simulink model "sampleModel7126_pp_1_1"  (R2018a)
settings: Solver=VariableStepAuto  StartTime=0.0  StopTime=10.0  RelTol=1e-3
undefined symbols (not defined in the file): DiscIntNeverNeededParam
libraries: simulink x367
(part 3 of 12)

== system sampleModel7126_pp_1_1/cfblk256 ==
  cfblk1 : Inport
  cfblk10 : Inport  Port=2
  Action Port : ActionPort  ActionType=else
  cfblk11 : Subsystem  TreatAsAtomicUnit=on
  cfblk12 : Subsystem  TreatAsAtomicUnit=on
  cfblk13 : Delay
  cfblk14 : Subsystem  TreatAsAtomicUnit=on
  cfblk15 : Delay
  cfblk3 : Subsystem  TreatAsAtomicUnit=on
  cfblk4 : DiscreteStateSpace  SampleTime=-1
  cfblk5 : DiscreteTransferFcn
  cfblk6 : simulink/Discrete/Transfer Fcn Real Zero  ZeroZ=0.75  ICPrevInput=0.0  DoSatur=off
      settings: SourceProductName=Simulink  SourceProductBaseCode=SL
  cfblk7 : simulink/Continuous/PID Controller  Controller=PID  TimeDomain=Discrete-time  SampleTime=-1  IntegratorMethod=Forward Euler  FilterMethod=Forward Euler  Form=Parallel  UseFilter=on  ControllerParametersSource=internal  P=1  I=1  D=0  N=100  InitialConditionSource=internal  InitialConditionForIntegrator=0  InitialConditionForFilter=0  ExternalReset=none  LimitOutput=off  UpperSaturationLimit=inf  LowerSaturationLimit=-inf  LinearizeAsGain=off  AntiWindupMode=none  Kb=1  TrackingMode=off  Kt=1  PParamMin=[]  PParamMax=[]  IParamMin=[]  IParamMax=[]  DParamMin=[]  DParamMax=[]  NParamMin=[]  NParamMax=[]  KbParamMin=[]  KbParamMax=[]  KtParamMin=[]  KtParamMax=[]  POutMin=[]  POutMax=[]  IOutMin=[]  IOutMax=[]  DOutMin=[]  DOutMax=[]  NOutMin=[]  NOutMax=[]  KbOutMin=[]  KbOutMax=[]  KtOutMin=[]  KtOutMax=[]  IntegratorOutMin=[]  IntegratorOutMax=[]  FilterOutMin=[]  FilterOutMax=[]  SumOutMin=[]  SumOutMax=[]  SumI1OutMin=[]  SumI1OutMax=[]  SumI2OutMin=[]  SumI2OutMax=[]  SumI3OutMin=[]  SumI3OutMax=[]  SumDOutMin=[]  SumDOutMax=[]  SaturationOutMin=[]  SaturationOutMax=[]  IntegratorContinuousStateAttributes=''  IntegratorStateMustResolveToSignalObject=off  IntegratorRTWStateStorageClass=Auto  FilterContinuousStateAttributes=''  FilterStateMustResolveToSignalObject=off  FilterRTWStateStorageClass=Auto  DifferentiatorICPrevScaledInput=0  DifferentiatorOutMin=[]  DifferentiatorOutMax=[]  FilterDiffOutCoefMin=[]  FilterDiffOutCoefMax=[]  SumDenOutMin=[]  SumDenOutMax=[]  SumNumOutMin=[]  SumNumOutMax=[]  ReciprocalOutMin=[]  ReciprocalOutMax=[]  DivideOutMin=[]  DivideOutMax=[]  TunerSelectOption=Transfer Function Based (PID Tuner App)
  cfblk8 : DiscreteFir
  cfblk9 : If  SampleTime=1
  cyemi_{359..361,368,373..382} (14 alike) : DataTypeConversion  OutDataTypeStr=double
  emi_1040 : Subsystem  TreatAsAtomicUnit=on
  emi_1042 : If  IfExpression=0 <= u1  SampleTime=[1 0]
  emi_1043 : DataTypeConversion  OutDataTypeStr=double
  emi_2146 : Subsystem  TreatAsAtomicUnit=on
  emi_2148 : If  IfExpression=0 <= u1  SampleTime=[1 0]
  emi_2149 : DataTypeConversion  OutDataTypeStr=double
  cfblk2 : Outport
  wires:
  cfblk1/1 -> cfblk2/1
  cfblk9/1 -> cfblk11/Action
  cfblk9/2 -> cfblk12/Action
  cyemi_359/1 -> cfblk11/1(cfblk1)
  cfblk13/1 -> cyemi_359/1, emi_1043/1
  cyemi_360/1 -> cfblk11/2(cfblk9)
  cfblk10/1 -> cyemi_360/1
  cyemi_361/1 -> cfblk11/3(cfblk10)
  cfblk12/3(cfblk8) -> cyemi_361/1
  cyemi_368/1 -> cfblk12/1(cfblk1)
  cfblk6/1 -> cyemi_368/1
  cyemi_373/1 -> cfblk13/1
  cfblk4/1 -> cyemi_373/1
  cfblk12/1(cfblk2) -> cyemi_374/1
  cyemi_375/1 -> cfblk15/1
  cfblk12/2(cfblk7) -> cyemi_375/1
  cfblk15/1 -> cyemi_376/1
  cyemi_377/1 -> cfblk4/1
  cfblk8/1 -> cyemi_377/1
  cyemi_378/1 -> cfblk5/1
  cfblk7/1 -> cyemi_378/1
  cyemi_379/1 -> cfblk6/1
  cfblk5/1 -> cyemi_379/1
  cyemi_380/1 -> cfblk7/1
  cyemi_381/1 -> cfblk8/1
  cfblk11/1(cfblk2) -> cyemi_381/1
  cyemi_382/1 -> cfblk9/1
  cyemi_376/1 -> cfblk3/1(emi_1038)
  cfblk3/1(emi_1039) -> cyemi_380/1, emi_2149/1
  emi_1042/1 -> cfblk3/Action
  emi_1042/2 -> emi_1040/Action
  emi_1043/1 -> emi_1042/1
  cyemi_374/1 -> cfblk14/1(emi_2144)
  cfblk14/1(emi_2145) -> cyemi_382/1
  emi_2148/1 -> cfblk14/Action
  emi_2148/2 -> emi_2146/Action
  emi_2149/1 -> emi_2148/1

== system sampleModel7126_pp_1_1/cfblk257 ==
  cfblk1 : Inport
  cfblk12 : Inport  Port=2
  cfblk13 : Inport  Port=3
  Action Port : ActionPort  ActionType=then
  cfblk10 : simulink/Discrete/Tapped Delay  vinit=0.0  samptime=-1  NumDelays=1  DelayOrder=Oldest  includeCurrent=off
  cfblk11 : simulink/Discrete/Difference  ICPrevInput=0.0  OutMin=[]  OutMax=[]  OutDataTypeStr=double  OutputDataTypeScalingMode=double  OutDataType=fixdt(1, 16)  OutScaling=2^-10  DoSatur=off
  cfblk3 : DiscreteFir
  cfblk4 : simulink/Continuous/PID Controller  Controller=PID  TimeDomain=Discrete-time  SampleTime=-1  IntegratorMethod=Forward Euler  FilterMethod=Forward Euler  Form=Parallel  UseFilter=on  ControllerParametersSource=internal  P=1  I=1  D=0  N=100  InitialConditionSource=internal  InitialConditionForIntegrator=0  InitialConditionForFilter=0  ExternalReset=none  LimitOutput=off  UpperSaturationLimit=inf  LowerSaturationLimit=-inf  LinearizeAsGain=off  AntiWindupMode=none  Kb=1  TrackingMode=off  Kt=1  PParamMin=[]  PParamMax=[]  IParamMin=[]  IParamMax=[]  DParamMin=[]  DParamMax=[]  NParamMin=[]  NParamMax=[]  KbParamMin=[]  KbParamMax=[]  KtParamMin=[]  KtParamMax=[]  POutMin=[]  POutMax=[]  IOutMin=[]  IOutMax=[]  DOutMin=[]  DOutMax=[]  NOutMin=[]  NOutMax=[]  KbOutMin=[]  KbOutMax=[]  KtOutMin=[]  KtOutMax=[]  IntegratorOutMin=[]  IntegratorOutMax=[]  FilterOutMin=[]  FilterOutMax=[]  SumOutMin=[]  SumOutMax=[]  SumI1OutMin=[]  SumI1OutMax=[]  SumI2OutMin=[]  SumI2OutMax=[]  SumI3OutMin=[]  SumI3OutMax=[]  SumDOutMin=[]  SumDOutMax=[]  SaturationOutMin=[]  SaturationOutMax=[]  IntegratorContinuousStateAttributes=''  IntegratorStateMustResolveToSignalObject=off  IntegratorRTWStateStorageClass=Auto  FilterContinuousStateAttributes=''  FilterStateMustResolveToSignalObject=off  FilterRTWStateStorageClass=Auto  DifferentiatorICPrevScaledInput=0  DifferentiatorOutMin=[]  DifferentiatorOutMax=[]  FilterDiffOutCoefMin=[]  FilterDiffOutCoefMax=[]  SumDenOutMin=[]  SumDenOutMax=[]  SumNumOutMin=[]  SumNumOutMax=[]  ReciprocalOutMin=[]  ReciprocalOutMax=[]  DivideOutMin=[]  DivideOutMax=[]  TunerSelectOption=Transfer Function Based (PID Tuner App)
  cfblk5 : simulink/Discrete/Transfer Fcn Real Zero  ZeroZ=0.75  ICPrevInput=0.0  DoSatur=off
      settings: SourceProductName=Simulink  SourceProductBaseCode=SL
  cfblk6 : simulink/Continuous/PID Controller  Controller=PID  TimeDomain=Discrete-time  SampleTime=-1  IntegratorMethod=Forward Euler  FilterMethod=Forward Euler  Form=Parallel  UseFilter=on  ControllerParametersSource=internal  P=1  I=1  D=0  N=100  InitialConditionSource=internal  InitialConditionForIntegrator=0  InitialConditionForFilter=0  ExternalReset=none  LimitOutput=off  UpperSaturationLimit=inf  LowerSaturationLimit=-inf  LinearizeAsGain=off  AntiWindupMode=none  Kb=1  TrackingMode=off  Kt=1  PParamMin=[]  PParamMax=[]  IParamMin=[]  IParamMax=[]  DParamMin=[]  DParamMax=[]  NParamMin=[]  NParamMax=[]  KbParamMin=[]  KbParamMax=[]  KtParamMin=[]  KtParamMax=[]  POutMin=[]  POutMax=[]  IOutMin=[]  IOutMax=[]  DOutMin=[]  DOutMax=[]  NOutMin=[]  NOutMax=[]  KbOutMin=[]  KbOutMax=[]  KtOutMin=[]  KtOutMax=[]  IntegratorOutMin=[]  IntegratorOutMax=[]  FilterOutMin=[]  FilterOutMax=[]  SumOutMin=[]  SumOutMax=[]  SumI1OutMin=[]  SumI1OutMax=[]  SumI2OutMin=[]  SumI2OutMax=[]  SumI3OutMin=[]  SumI3OutMax=[]  SumDOutMin=[]  SumDOutMax=[]  SaturationOutMin=[]  SaturationOutMax=[]  IntegratorContinuousStateAttributes=''  IntegratorStateMustResolveToSignalObject=off  IntegratorRTWStateStorageClass=Auto  FilterContinuousStateAttributes=''  FilterStateMustResolveToSignalObject=off  FilterRTWStateStorageClass=Auto  DifferentiatorICPrevScaledInput=0  DifferentiatorOutMin=[]  DifferentiatorOutMax=[]  FilterDiffOutCoefMin=[]  FilterDiffOutCoefMax=[]  SumDenOutMin=[]  SumDenOutMax=[]  SumNumOutMin=[]  SumNumOutMax=[]  ReciprocalOutMin=[]  ReciprocalOutMax=[]  DivideOutMin=[]  DivideOutMax=[]  TunerSelectOption=Transfer Function Based (PID Tuner App)
  cfblk7 : Subsystem  TreatAsAtomicUnit=on
  cfblk8 : UnitDelay  SampleTime=-1
  cfblk9 : Subsystem  TreatAsAtomicUnit=on
  cyemi_{386..394} (9 alike) : DataTypeConversion  OutDataTypeStr=double
  emi_1634 : Subsystem  TreatAsAtomicUnit=on
  emi_1636 : If  IfExpression=Inf <= u1  SampleTime=[1 0]
  emi_1637 : DataTypeConversion  OutDataTypeStr=double
  emi_727 : Subsystem  TreatAsAtomicUnit=on
  emi_729 : If  IfExpression=Inf <= u1  SampleTime=[1 0]
  emi_730 : DataTypeConversion  OutDataTypeStr=double
  cfblk2 : Outport
  cfblk14 : Outport  Port=2
  wires:
  cfblk3/1 -> cfblk14/1, emi_730/1
  cfblk11/1 -> cfblk2/1
  cyemi_386/1 -> cfblk10/1
  cfblk1/1 -> cyemi_386/1
  cyemi_387/1 -> cfblk11/1
  cfblk6/1 -> cyemi_387/1
  cyemi_388/1 -> cfblk3/1
  cfblk8/1 -> cyemi_388/1
  cyemi_389/1 -> cfblk4/1
  cfblk12/1 -> cyemi_389/1
  cyemi_390/1 -> cfblk5/1
  cyemi_391/1 -> cfblk6/1
  cfblk4/1 -> cyemi_392/1
  cyemi_393/1 -> cfblk8/1
  cfblk5/1 -> cyemi_393/1
  cfblk10/1 -> cyemi_394/1, emi_1637/1
  cyemi_394/1 -> cfblk9/1(emi_725)
  cfblk9/1(emi_726) -> cyemi_391/1
  emi_729/1 -> cfblk9/Action
  emi_729/2 -> emi_727/Action
  emi_730/1 -> emi_729/1
  cyemi_392/1 -> cfblk7/1(emi_1632)
  cfblk7/1(emi_1633) -> cyemi_390/1
  emi_1636/1 -> cfblk7/Action
  emi_1636/2 -> emi_1634/Action
  emi_1637/1 -> emi_1636/1

== system sampleModel7126_pp_1_1/cfblk258 ==
  cfblk1 : Inport
  cfblk8 : Inport  Port=2
  cfblk9 : Inport  Port=3
  cfblk10 : Inport  Port=4
  Action Port : ActionPort  ActionType=else
  cfblk11 : Delay
  cfblk3 : UnitDelay  SampleTime=-1
  cfblk4 : DiscreteFir
  cfblk5 : Subsystem  TreatAsAtomicUnit=on
  cfblk6 : Delay  ShowEnablePort=on
      settings: InputPortMap=u0,e6
  cfblk7 : simulink/Continuous/PID Controller (2DOF)  Controller=PID  TimeDomain=Discrete-time  SampleTime=-1  IntegratorMethod=Forward Euler  FilterMethod=Forward Euler  Form=Parallel  UseFilter=on  ControllerParametersSource=internal  P=1  I=1  D=0  N=100  b=1  c=1  InitialConditionSource=internal  InitialConditionForIntegrator=0  InitialConditionForFilter=0  ExternalReset=none  LimitOutput=off  UpperSaturationLimit=inf  LowerSaturationLimit=-inf  LinearizeAsGain=off  AntiWindupMode=none  Kb=1  TrackingMode=off  Kt=1  PParamMin=[]  PParamMax=[]  IParamMin=[]  IParamMax=[]  DParamMin=[]  DParamMax=[]  NParamMin=[]  NParamMax=[]  bParamMin=[]  bParamMax=[]  cParamMin=[]  cParamMax=[]  KbParamMin=[]  KbParamMax=[]  KtParamMin=[]  KtParamMax=[]  POutMin=[]  POutMax=[]  IOutMin=[]  IOutMax=[]  DOutMin=[]  DOutMax=[]  NOutMin=[]  NOutMax=[]  bOutMin=[]  bOutMax=[]  cOutMin=[]  cOutMax=[]  KbOutMin=[]  KbOutMax=[]  KtOutMin=[]  KtOutMax=[]  IntegratorOutMin=[]  IntegratorOutMax=[]  FilterOutMin=[]  FilterOutMax=[]  SumOutMin=[]  SumOutMax=[]  Sum1OutMin=[]  Sum1OutMax=[]  Sum2OutMin=[]  Sum2OutMax=[]  Sum3OutMin=[]  Sum3OutMax=[]  SumI1OutMin=[]  SumI1OutMax=[]  SumI2OutMin=[]  SumI2OutMax=[]  SumI3OutMin=[]  SumI3OutMax=[]  SumDOutMin=[]  SumDOutMax=[]  SaturationOutMin=[]  SaturationOutMax=[]  IntegratorContinuousStateAttributes=''  IntegratorStateMustResolveToSignalObject=off  IntegratorRTWStateStorageClass=Auto  FilterContinuousStateAttributes=''  FilterStateMustResolveToSignalObject=off  FilterRTWStateStorageClass=Auto  DifferentiatorICPrevScaledInput=0  DifferentiatorOutMin=[]  DifferentiatorOutMax=[]  FilterDiffOutCoefMin=[]  FilterDiffOutCoefMax=[]  SumDenOutMin=[]  SumDenOutMax=[]  SumNumOutMin=[]  SumNumOutMax=[]  ReciprocalOutMin=[]  ReciprocalOutMax=[]  DivideOutMin=[]  DivideOutMax=[]  TunerSelectOption=Transfer Function Based (PID Tuner App)
  cyemi_{399..406} (8 alike) : DataTypeConversion  OutDataTypeStr=double
  emi_1343 : Subsystem  TreatAsAtomicUnit=on
  emi_1345 : If  IfExpression=0 <= u1  SampleTime=[1 0]
  emi_1346 : DataTypeConversion  OutDataTypeStr=double
  cfblk2 : Outport
  wires:
  cfblk10/1 -> cfblk2/1
  cyemi_399/1 -> cfblk11/1
  cyemi_400/1 -> cfblk3/1
  cfblk9/1 -> cyemi_400/1
  cyemi_401/1 -> cfblk4/1
  cfblk8/1 -> cyemi_401/1
  cfblk7/1 -> cyemi_402/1
  cyemi_403/1 -> cfblk6/1
  cfblk11/1 -> cyemi_403/1
  cyemi_404/1 -> cfblk6/2
  cfblk3/1 -> cyemi_404/1, emi_1346/1
  cyemi_405/1 -> cfblk7/1
  cfblk4/1 -> cyemi_405/1
  cyemi_406/1 -> cfblk7/2
  cfblk6/1 -> cyemi_406/1
  cyemi_402/1 -> cfblk5/1(emi_1341)
  cfblk5/1(emi_1342) -> cyemi_399/1
  emi_1345/1 -> cfblk5/Action
  emi_1345/2 -> emi_1343/Action
  emi_1346/1 -> emi_1345/1

== system sampleModel7126_pp_1_1/cfblk259 ==
  cfblk1 : Inport
  Action Port : ActionPort  ActionType=then
  cfblk10 : Subsystem  TreatAsAtomicUnit=on
  cfblk11 : Subsystem  TreatAsAtomicUnit=on
  cfblk12 : Delay
  cfblk13 : Subsystem  TreatAsAtomicUnit=on
  cfblk3 : Subsystem  TreatAsAtomicUnit=on
  cfblk4 : Subsystem  TreatAsAtomicUnit=on
  cfblk5 : simulink/Discrete/Tapped Delay  vinit=0.0  samptime=-1  NumDelays=1  DelayOrder=Oldest  includeCurrent=off
  cfblk6 : Subsystem  TreatAsAtomicUnit=on
  cfblk7 : If  SampleTime=1
  cfblk9 : Subsystem  TreatAsAtomicUnit=on
  cyemi_{408..411,421..431} (15 alike) : DataTypeConversion  OutDataTypeStr=double
  emi_1161 : Subsystem  TreatAsAtomicUnit=on
  emi_{62,560,1163,1774} (4 alike) : If  IfExpression=Inf <= u1  SampleTime=[1 0]
  emi_{48,63,561,1164,1775} (5 alike) : DataTypeConversion  OutDataTypeStr=double
  emi_1772 : Subsystem  TreatAsAtomicUnit=on
  emi_45 : Subsystem  TreatAsAtomicUnit=on
  emi_47 : If  IfExpression=Inf <= u1
  emi_558 : Subsystem  TreatAsAtomicUnit=on
  emi_60 : Subsystem  TreatAsAtomicUnit=on
  cfblk2 : Outport
  cfblk8 : Outport  Port=2
  wires:
  cfblk5/1 -> cfblk8/1, cyemi_421/1, emi_63/1, emi_1775/1
  cfblk7/1 -> cfblk9/Action
  cfblk7/2 -> cfblk10/Action
  cyemi_408/1 -> cfblk10/1(cfblk1)
  cfblk1/1 -> cyemi_408/1
  cyemi_409/1 -> cfblk10/2(cfblk10)
  cyemi_410/1 -> cfblk10/3(cfblk11)
  cyemi_411/1 -> cfblk10/4(cfblk12)
  cyemi_422/1 -> cfblk12/1
  cfblk9/1(cfblk2) -> cyemi_422/1
  cfblk9/2(cfblk12) -> cyemi_423/1
  cfblk9/3(cfblk13) -> cyemi_424/1, cyemi_425/1
  cyemi_427/1 -> cfblk5/1
  cfblk10/1(cfblk2) -> cyemi_427/1
  cyemi_429/1 -> cfblk7/1
  cfblk12/1 -> cyemi_429/1
  cyemi_430/1 -> cfblk9/1(cfblk1)
  cyemi_431/1 -> cfblk9/2(cfblk11)
  cyemi_421/1 -> cfblk11/1(emi_43)
  cfblk11/1(emi_44) -> cyemi_411/1, emi_561/1, emi_1164/1
  emi_47/1 -> cfblk11/Action
  emi_47/2 -> emi_45/Action
  emi_48/1 -> emi_47/1
  cyemi_423/1 -> cfblk13/1(emi_58)
  cfblk13/1(emi_59) -> cyemi_428/1
  emi_62/1 -> cfblk13/Action
  emi_62/2 -> emi_60/Action
  emi_63/1 -> emi_62/1
  cyemi_428/1 -> cfblk6/1(emi_556)
  cfblk6/1(emi_557) -> cyemi_431/1, cyemi_430/1, cyemi_426/1, cyemi_410/1
  emi_560/1 -> cfblk6/Action
  emi_560/2 -> emi_558/Action
  emi_561/1 -> emi_560/1
  cyemi_426/1 -> cfblk4/1(emi_1159)
  cfblk4/1(emi_1160) -> emi_48/1, cyemi_409/1
  emi_1163/1 -> cfblk4/Action
  emi_1163/2 -> emi_1161/Action
  emi_1164/1 -> emi_1163/1
  cyemi_424/1 -> cfblk3/1(emi_1769)
  cyemi_425/1 -> cfblk3/2(emi_1770)
  cfblk3/1(emi_1771) -> cfblk2/1
  emi_1774/1 -> cfblk3/Action
  emi_1774/2 -> emi_1772/Action
  emi_1775/1 -> emi_1774/1

== system sampleModel7126_pp_1_1/cfblk26 ==
  emi_1504 : Inport
  Action Port : ActionPort  ActionType=then
  cfblk26 : simulink/Discrete/Transfer Fcn First Order  PoleZ=0.95  ICPrevOutput=0.0  DoSatur=off
      settings: SourceProductName=Simulink
  emi_1505 : Outport
  wires:
  emi_1504/1 -> cfblk26/1
  cfblk26/1 -> emi_1505/1

== system sampleModel7126_pp_1_1/cfblk260 ==
  cfblk1 : Inport
  cfblk9 : Inport  Port=2
  Action Port : ActionPort  ActionType=else
  cfblk13 : Delay
  cfblk3 : simulink/Discrete/Transfer Fcn Real Zero  ZeroZ=0.75  ICPrevInput=0.0  DoSatur=off
      settings: SourceProductName=Simulink  SourceProductBaseCode=SL
  cfblk4 : Subsystem  TreatAsAtomicUnit=on
  cfblk5 : Subsystem  TreatAsAtomicUnit=on
  cfblk6 : Subsystem  TreatAsAtomicUnit=on
  cfblk7 : Delay  DelayLengthSource=Input port
      settings: InputPortMap=u0,p1
  cfblk8 : simulink/Discrete/Transfer Fcn Lead or Lag  PoleZ=0.95  ZeroZ=0.75  ICPrevOutput=0.0  ICPrevInput=0.0  DoSatur=off
      settings: SourceProductName=Simulink  SourceProductBaseCode=SL
  cyemi_{449..456} (8 alike) : DataTypeConversion  OutDataTypeStr=double
  emi_10 : Subsystem  TreatAsAtomicUnit=on
  emi_12 : If  IfExpression=0 <= u1  SampleTime=[1 0]
  emi_13 : DataTypeConversion  OutDataTypeStr=double
  emi_254 : Subsystem  TreatAsAtomicUnit=on
  emi_256 : If  IfExpression=0 <= u1  SampleTime=[1 0]
  emi_257 : DataTypeConversion  OutDataTypeStr=double
  emi_410 : Subsystem  TreatAsAtomicUnit=on
  emi_412 : If  IfExpression=0 <= u1  SampleTime=[1 0]
  emi_413 : DataTypeConversion  OutDataTypeStr=double
  cfblk2 : Outport
  cfblk10 : Outport  Port=2
  cfblk11 : Outport  Port=3
  cfblk12 : Outport  Port=4
  wires:
  cfblk8/1 -> cfblk10/1
  cfblk3/1 -> cyemi_451/1, cyemi_452/1
  cfblk9/1 -> cfblk11/1, cfblk2/1
  cyemi_449/1 -> cfblk13/1
  cyemi_450/1 -> cfblk3/1
  cfblk13/1 -> cyemi_450/1, emi_13/1, emi_257/1
  cyemi_454/1 -> cfblk7/1
  cyemi_455/1 -> cfblk7/2
  cfblk1/1 -> cyemi_455/1
  cyemi_456/1 -> cfblk8/1
  cfblk7/1 -> cyemi_456/1
  cyemi_452/1 -> cfblk5/1(emi_8)
  cfblk5/1(emi_9) -> cyemi_449/1, emi_413/1
  emi_12/1 -> cfblk5/Action
  emi_12/2 -> emi_10/Action
  emi_13/1 -> emi_12/1
  cyemi_451/1 -> cfblk4/1(emi_252)
  cfblk4/1(emi_253) -> cyemi_453/1, cfblk12/1
  emi_256/1 -> cfblk4/Action
  emi_256/2 -> emi_254/Action
  emi_257/1 -> emi_256/1
  cyemi_453/1 -> cfblk6/1(emi_408)
  cfblk6/1(emi_409) -> cyemi_454/1
  emi_412/1 -> cfblk6/Action
  emi_412/2 -> emi_410/Action
  emi_413/1 -> emi_412/1

== system sampleModel7126_pp_1_1/cfblk261 ==
  cfblk1 : Inport
  Action Port : ActionPort  ActionType=then
  cfblk10 : simulink/Discrete/Difference  ICPrevInput=0.0  OutMin=[]  OutMax=[]  OutDataTypeStr=double  OutputDataTypeScalingMode=double  OutDataType=fixdt(1, 16)  OutScaling=2^-10  DoSatur=off
  cfblk11 : If  SampleTime=1
  cfblk13 : Subsystem  TreatAsAtomicUnit=on
  cfblk14 : Subsystem  TreatAsAtomicUnit=on
  cfblk15 : Subsystem  TreatAsAtomicUnit=on
  cfblk16 : Delay
  cfblk17 : Delay
  cfblk3 : simulink/Discrete/Difference  ICPrevInput=0.0  OutMin=[]  OutMax=[]  OutDataTypeStr=double  OutputDataTypeScalingMode=double  OutDataType=fixdt(1, 16)  OutScaling=2^-10  DoSatur=off
  cfblk4 : DiscreteFilter
  cfblk5 : DiscreteTransferFcn
  cfblk6 : simulink/Continuous/PID Controller (2DOF)  Controller=PID  TimeDomain=Discrete-time  SampleTime=-1  IntegratorMethod=Forward Euler  FilterMethod=Forward Euler  Form=Parallel  UseFilter=on  ControllerParametersSource=internal  P=1  I=1  D=0  N=100  b=1  c=1  InitialConditionSource=internal  InitialConditionForIntegrator=0  InitialConditionForFilter=0  ExternalReset=none  LimitOutput=off  UpperSaturationLimit=inf  LowerSaturationLimit=-inf  LinearizeAsGain=off  AntiWindupMode=none  Kb=1  TrackingMode=off  Kt=1  PParamMin=[]  PParamMax=[]  IParamMin=[]  IParamMax=[]  DParamMin=[]  DParamMax=[]  NParamMin=[]  NParamMax=[]  bParamMin=[]  bParamMax=[]  cParamMin=[]  cParamMax=[]  KbParamMin=[]  KbParamMax=[]  KtParamMin=[]  KtParamMax=[]  POutMin=[]  POutMax=[]  IOutMin=[]  IOutMax=[]  DOutMin=[]  DOutMax=[]  NOutMin=[]  NOutMax=[]  bOutMin=[]  bOutMax=[]  cOutMin=[]  cOutMax=[]  KbOutMin=[]  KbOutMax=[]  KtOutMin=[]  KtOutMax=[]  IntegratorOutMin=[]  IntegratorOutMax=[]  FilterOutMin=[]  FilterOutMax=[]  SumOutMin=[]  SumOutMax=[]  Sum1OutMin=[]  Sum1OutMax=[]  Sum2OutMin=[]  Sum2OutMax=[]  Sum3OutMin=[]  Sum3OutMax=[]  SumI1OutMin=[]  SumI1OutMax=[]  SumI2OutMin=[]  SumI2OutMax=[]  SumI3OutMin=[]  SumI3OutMax=[]  SumDOutMin=[]  SumDOutMax=[]  SaturationOutMin=[]  SaturationOutMax=[]  IntegratorContinuousStateAttributes=''  IntegratorStateMustResolveToSignalObject=off  IntegratorRTWStateStorageClass=Auto  FilterContinuousStateAttributes=''  FilterStateMustResolveToSignalObject=off  FilterRTWStateStorageClass=Auto  DifferentiatorICPrevScaledInput=0  DifferentiatorOutMin=[]  DifferentiatorOutMax=[]  FilterDiffOutCoefMin=[]  FilterDiffOutCoefMax=[]  SumDenOutMin=[]  SumDenOutMax=[]  SumNumOutMin=[]  SumNumOutMax=[]  ReciprocalOutMin=[]  ReciprocalOutMax=[]  DivideOutMin=[]  DivideOutMax=[]  TunerSelectOption=Transfer Function Based (PID Tuner App)
  cfblk7 : Delay  ShowEnablePort=on
      settings: InputPortMap=u0,e6
  cfblk8 : Subsystem  TreatAsAtomicUnit=on
  cfblk9 : Subsystem  TreatAsAtomicUnit=on
  cyemi_{458..460,469..470,473..484} (17 alike) : DataTypeConversion  OutDataTypeStr=double
  emi_1966 : Subsystem  TreatAsAtomicUnit=on
  emi_1968 : If  IfExpression=0 <= u1  SampleTime=[1 0]
  emi_1969 : DataTypeConversion  OutDataTypeStr=double
  emi_1973 : Subsystem  TreatAsAtomicUnit=on
  emi_1975 : If  IfExpression=0 <= u1  SampleTime=[1 0]
  emi_1976 : DataTypeConversion  OutDataTypeStr=double
  emi_2196 : Subsystem  TreatAsAtomicUnit=on
  emi_2198 : If  IfExpression=0 <= u1  SampleTime=[0.1 0]
  emi_2199 : DataTypeConversion  OutDataTypeStr=double
  cfblk2 : Outport
  cfblk12 : Outport  Port=2
  wires:
  cfblk7/1 -> cyemi_459/1, cyemi_476/1
  cfblk13/1(cfblk2) -> cyemi_470/1, cyemi_479/1
  cfblk14/1(cfblk2) -> cfblk12/1
  cfblk11/1 -> cfblk13/Action
  cfblk11/2 -> cfblk14/Action
  cyemi_458/1 -> cfblk10/1
  cfblk14/3(cfblk7) -> cyemi_458/1
  cyemi_459/1 -> cfblk11/1
  cyemi_460/1 -> cfblk13/1(cfblk1)
  cfblk3/1 -> cyemi_460/1
  cyemi_469/1 -> cfblk14/1(cfblk1)
  cfblk16/1 -> cyemi_469/1
  cyemi_470/1 -> cfblk14/2(cfblk5)
  cyemi_474/1 -> cfblk16/1
  cfblk4/1 -> cyemi_474/1, emi_1969/1, emi_1976/1, emi_2199/1
  cyemi_475/1 -> cfblk17/1
  cfblk10/1 -> cyemi_475/1
  cyemi_476/1 -> cfblk3/1
  cyemi_477/1 -> cfblk4/1
  cfblk14/2(cfblk6) -> cyemi_477/1
  cyemi_478/1 -> cfblk5/1
  cyemi_479/1 -> cfblk6/1
  cyemi_480/1 -> cfblk6/2
  cyemi_481/1 -> cfblk7/1
  cfblk1/1 -> cyemi_481/1
  cyemi_482/1 -> cfblk7/2
  cfblk17/1 -> cyemi_482/1
  cfblk6/1 -> cyemi_483/1
  cfblk5/1 -> cyemi_484/1
  cyemi_473/1 -> cfblk15/1(emi_1964)
  cfblk15/1(emi_1965) -> cyemi_480/1
  emi_1968/1 -> cfblk15/Action
  emi_1968/2 -> emi_1966/Action
  emi_1969/1 -> emi_1968/1
  cyemi_483/1 -> cfblk8/1(emi_1971)
  cfblk8/1(emi_1972) -> cyemi_478/1, cyemi_473/1
  emi_1975/1 -> cfblk8/Action
  emi_1975/2 -> emi_1973/Action
  emi_1976/1 -> emi_1975/1
  cyemi_484/1 -> cfblk9/1(emi_2194)
  cfblk9/1(emi_2195) -> cfblk2/1
  emi_2198/1 -> cfblk9/Action
  emi_2198/2 -> emi_2196/Action
  emi_2199/1 -> emi_2198/1

== system sampleModel7126_pp_1_1/cfblk262 ==
  cfblk1 : Inport
  cfblk9 : Inport  Port=2
  Action Port : ActionPort  ActionType=else
  cfblk11 : Delay
  cfblk3 : simulink/Continuous/PID Controller  Controller=PID  TimeDomain=Discrete-time  SampleTime=-1  IntegratorMethod=Forward Euler  FilterMethod=Forward Euler  Form=Parallel  UseFilter=on  ControllerParametersSource=internal  P=1  I=1  D=0  N=100  InitialConditionSource=internal  InitialConditionForIntegrator=0  InitialConditionForFilter=0  ExternalReset=none  LimitOutput=off  UpperSaturationLimit=inf  LowerSaturationLimit=-inf  LinearizeAsGain=off  AntiWindupMode=none  Kb=1  TrackingMode=off  Kt=1  PParamMin=[]  PParamMax=[]  IParamMin=[]  IParamMax=[]  DParamMin=[]  DParamMax=[]  NParamMin=[]  NParamMax=[]  KbParamMin=[]  KbParamMax=[]  KtParamMin=[]  KtParamMax=[]  POutMin=[]  POutMax=[]  IOutMin=[]  IOutMax=[]  DOutMin=[]  DOutMax=[]  NOutMin=[]  NOutMax=[]  KbOutMin=[]  KbOutMax=[]  KtOutMin=[]  KtOutMax=[]  IntegratorOutMin=[]  IntegratorOutMax=[]  FilterOutMin=[]  FilterOutMax=[]  SumOutMin=[]  SumOutMax=[]  SumI1OutMin=[]  SumI1OutMax=[]  SumI2OutMin=[]  SumI2OutMax=[]  SumI3OutMin=[]  SumI3OutMax=[]  SumDOutMin=[]  SumDOutMax=[]  SaturationOutMin=[]  SaturationOutMax=[]  IntegratorContinuousStateAttributes=''  IntegratorStateMustResolveToSignalObject=off  IntegratorRTWStateStorageClass=Auto  FilterContinuousStateAttributes=''  FilterStateMustResolveToSignalObject=off  FilterRTWStateStorageClass=Auto  DifferentiatorICPrevScaledInput=0  DifferentiatorOutMin=[]  DifferentiatorOutMax=[]  FilterDiffOutCoefMin=[]  FilterDiffOutCoefMax=[]  SumDenOutMin=[]  SumDenOutMax=[]  SumNumOutMin=[]  SumNumOutMax=[]  ReciprocalOutMin=[]  ReciprocalOutMax=[]  DivideOutMin=[]  DivideOutMax=[]  TunerSelectOption=Transfer Function Based (PID Tuner App)
  cfblk4 : Subsystem  TreatAsAtomicUnit=on
  cfblk5 : Subsystem  TreatAsAtomicUnit=on
  cfblk6 : Subsystem  TreatAsAtomicUnit=on
  cfblk7 : DiscreteFilter
  cfblk8 : Delay
  cyemi_{487..494} (8 alike) : DataTypeConversion  OutDataTypeStr=double
  emi_332 : Subsystem  TreatAsAtomicUnit=on
  emi_334 : If  IfExpression=0 <= u1  SampleTime=[1 0]
  emi_335 : DataTypeConversion  OutDataTypeStr=double
  emi_476 : Subsystem  TreatAsAtomicUnit=on
  emi_478 : If  IfExpression=0 <= u1  SampleTime=[1 0]
  emi_479 : DataTypeConversion  OutDataTypeStr=double
  emi_53 : Subsystem  TreatAsAtomicUnit=on
  emi_55 : If  IfExpression=0 <= u1  SampleTime=[1 0]
  emi_56 : DataTypeConversion  OutDataTypeStr=double
  cfblk2 : Outport
  cfblk10 : Outport  Port=2
  wires:
  cfblk7/1 -> cfblk2/1
  cfblk9/1 -> cfblk10/1
  cfblk8/1 -> cyemi_487/1, cyemi_488/1, emi_335/1
  cyemi_487/1 -> cfblk11/1
  cyemi_488/1 -> cfblk3/1
  cfblk1/1 -> cyemi_489/1
  cfblk11/1 -> cyemi_491/1, emi_56/1, emi_479/1
  cyemi_493/1 -> cfblk7/1
  cfblk3/1 -> cyemi_493/1
  cyemi_494/1 -> cfblk8/1
  cyemi_490/1 -> cfblk5/1(emi_50)
  cyemi_491/1 -> cfblk5/2(emi_51)
  cfblk5/1(emi_52) -> cyemi_494/1
  emi_55/1 -> cfblk5/Action
  emi_55/2 -> emi_53/Action
  emi_56/1 -> emi_55/1
  cyemi_492/1 -> cfblk6/1(emi_330)
  cfblk6/1(emi_331) -> cyemi_490/1
  emi_334/1 -> cfblk6/Action
  emi_334/2 -> emi_332/Action
  emi_335/1 -> emi_334/1
  cyemi_489/1 -> cfblk4/1(emi_474)
  cfblk4/1(emi_475) -> cyemi_492/1
  emi_478/1 -> cfblk4/Action
  emi_478/2 -> emi_476/Action
  emi_479/1 -> emi_478/1

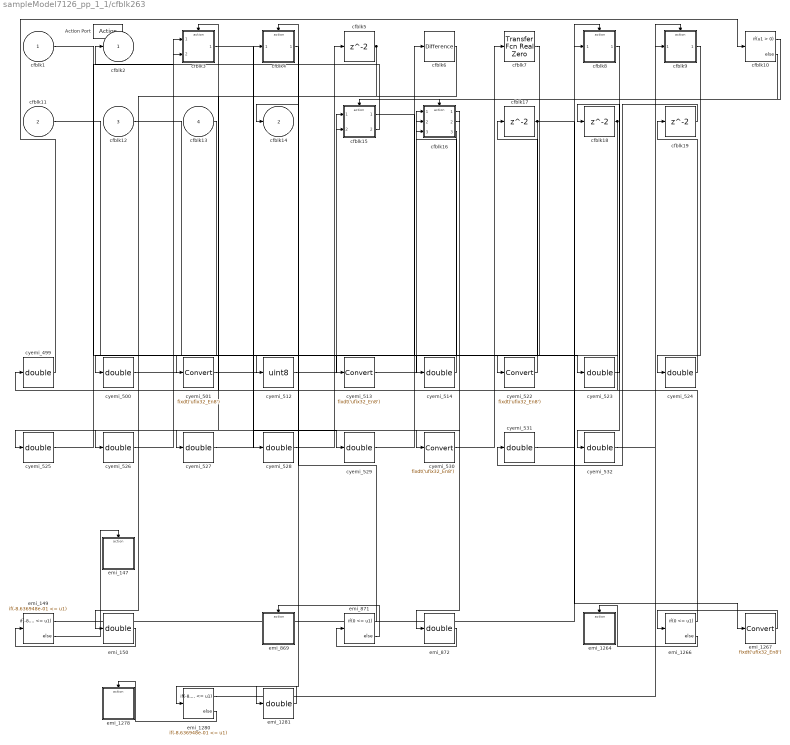
== system sampleModel7126_pp_1_1/cfblk263 ==
  cfblk1 : Inport
  cfblk11 : Inport  Port=2
  cfblk12 : Inport  Port=3
  cfblk13 : Inport  Port=4
  Action Port : ActionPort  ActionType=then
  cfblk10 : If  SampleTime=1
  cfblk15 : Subsystem  TreatAsAtomicUnit=on
  cfblk16 : Subsystem  TreatAsAtomicUnit=on
  cfblk{5,17..19} (4 alike) : Delay
  cfblk3 : Subsystem  TreatAsAtomicUnit=on
  cfblk4 : Subsystem  TreatAsAtomicUnit=on
  cfblk6 : simulink/Discrete/Difference  ICPrevInput=0.0  OutMin=[]  OutMax=[]  OutDataTypeStr=double  OutputDataTypeScalingMode=double  OutDataType=fixdt(1, 16)  OutScaling=2^-10  DoSatur=off
  cfblk7 : simulink/Discrete/Transfer Fcn Real Zero  ZeroZ=0.75  ICPrevInput=0.0  DoSatur=off
      settings: SourceProductName=Simulink  SourceProductBaseCode=SL
  cfblk8 : Subsystem  TreatAsAtomicUnit=on
  cfblk9 : Subsystem  TreatAsAtomicUnit=on
  cyemi_{499..500,514,523..529,531..532} (12 alike) : DataTypeConversion  OutDataTypeStr=double
  cyemi_{501,513,522,530} (4 alike) : DataTypeConversion  OutDataTypeStr=fixdt('ufix32_En8')
  cyemi_512 : DataTypeConversion  OutDataTypeStr=uint8
  emi_1264 : Subsystem  TreatAsAtomicUnit=on
  emi_1266 : If  IfExpression=0 <= u1  SampleTime=[1 0]
  emi_1267 : DataTypeConversion  OutDataTypeStr=fixdt('ufix32_En8')
  emi_1278 : Subsystem  TreatAsAtomicUnit=on
  emi_1280 : If  IfExpression=-8.636948e-01 <= u1  SampleTime=[1 0]
  emi_1281 : DataTypeConversion  OutDataTypeStr=double
  emi_147 : Subsystem  TreatAsAtomicUnit=on
  emi_149 : If  IfExpression=-8.636948e-01 <= u1  SampleTime=[1 0]
  emi_150 : DataTypeConversion  OutDataTypeStr=double
  emi_869 : Subsystem  TreatAsAtomicUnit=on
  emi_871 : If  IfExpression=0 <= u1  SampleTime=[1 0]
  emi_872 : DataTypeConversion  OutDataTypeStr=double
  cfblk2 : Outport
  cfblk14 : Outport  Port=2
  wires:
  cfblk15/2(cfblk12) -> cfblk2/1
  cfblk10/1 -> cfblk15/Action
  cfblk10/2 -> cfblk16/Action
  cyemi_499/1 -> cfblk10/1
  cfblk18/1 -> cyemi_499/1, emi_872/1
  cyemi_500/1 -> cfblk15/1(cfblk1)
  cfblk13/1 -> cyemi_500/1
  cyemi_501/1 -> cfblk15/2(cfblk11)
  cfblk16/3(cfblk13) -> cyemi_501/1
  cyemi_512/1 -> cfblk16/1(cfblk1)
  cfblk1/1 -> cyemi_512/1
  cyemi_513/1 -> cfblk16/2(cfblk10)
  cfblk17/1 -> cyemi_513/1, emi_1267/1
  cyemi_514/1 -> cfblk16/3(cfblk11)
  cfblk11/1 -> cyemi_514/1
  cyemi_522/1 -> cfblk17/1
  cfblk7/1 -> cyemi_522/1
  cyemi_523/1 -> cfblk18/1
  cfblk15/1(cfblk2) -> cyemi_523/1
  cyemi_524/1 -> cfblk19/1
  cfblk16/1(cfblk2) -> cyemi_525/1
  cfblk5/1 -> cyemi_526/1, emi_150/1, emi_1281/1
  cfblk6/1 -> cyemi_527/1
  cyemi_528/1 -> cfblk5/1
  cfblk12/1 -> cyemi_528/1
  cyemi_529/1 -> cfblk6/1
  cyemi_530/1 -> cfblk7/1
  cfblk16/2(cfblk12) -> cyemi_530/1
  cfblk19/1 -> cyemi_531/1
  cyemi_531/1 -> cfblk8/1(emi_145)
  cfblk8/1(emi_146) -> cyemi_532/1
  emi_149/1 -> cfblk8/Action
  emi_149/2 -> emi_147/Action
  emi_150/1 -> emi_149/1
  cyemi_527/1 -> cfblk4/1(emi_867)
  cfblk4/1(emi_868) -> cfblk14/1
  emi_871/1 -> cfblk4/Action
  emi_871/2 -> emi_869/Action
  emi_872/1 -> emi_871/1
  cyemi_525/1 -> cfblk3/1(emi_1261)
  cyemi_526/1 -> cfblk3/2(emi_1262)
  cfblk3/1(emi_1263) -> cyemi_529/1
  emi_1266/1 -> cfblk3/Action
  emi_1266/2 -> emi_1264/Action
  emi_1267/1 -> emi_1266/1
  cyemi_532/1 -> cfblk9/1(emi_1276)
  cfblk9/1(emi_1277) -> cyemi_524/1
  emi_1280/1 -> cfblk9/Action
  emi_1280/2 -> emi_1278/Action
  emi_1281/1 -> emi_1280/1

== system sampleModel7126_pp_1_1/cfblk264 ==
  cfblk1 : Inport
  cfblk12 : Inport  Port=2
  Action Port : ActionPort  ActionType=else
  cfblk10 : Subsystem  TreatAsAtomicUnit=on
  cfblk11 : Delay  DelayLengthSource=Input port
      settings: InputPortMap=u0,p1
  cfblk15 : Delay
  cfblk16 : Delay
  cfblk3 : DiscreteFir
  cfblk4 : DiscreteZeroPole  Poles=[0 0.5]  Gain=1  SampleTime=-1
  cfblk5 : Subsystem  TreatAsAtomicUnit=on
  cfblk6 : DiscreteTransferFcn
  cfblk7 : Subsystem  TreatAsAtomicUnit=on
  cfblk8 : Subsystem  TreatAsAtomicUnit=on
  cfblk9 : Subsystem  TreatAsAtomicUnit=on
  cyemi_{535..547} (13 alike) : DataTypeConversion  OutDataTypeStr=double
  emi_{236,420,1000,1723,1860} (5 alike) : DataTypeConversion  OutDataTypeStr=double
  emi_1720 : Subsystem  TreatAsAtomicUnit=on
  emi_{235,999,1722,1859} (4 alike) : If  IfExpression=Inf <= u1  SampleTime=[1 0]
  emi_1857 : Subsystem  TreatAsAtomicUnit=on
  emi_233 : Subsystem  TreatAsAtomicUnit=on
  emi_417 : Subsystem  TreatAsAtomicUnit=on
  emi_419 : If  IfExpression=Inf <= u1
  emi_997 : Subsystem  TreatAsAtomicUnit=on
  cfblk2 : Outport
  cfblk13 : Outport  Port=2
  cfblk14 : Outport  Port=3
  wires:
  cfblk6/1 -> cfblk2/1, cyemi_538/1
  cfblk11/1 -> cfblk13/1, emi_1000/1, emi_1723/1
  cyemi_536/1 -> cfblk11/1
  cfblk12/1 -> cyemi_536/1
  cyemi_537/1 -> cfblk11/2
  cyemi_538/1 -> cfblk15/1
  cyemi_539/1 -> cfblk16/1
  cyemi_540/1 -> cfblk3/1
  cfblk4/1 -> cyemi_540/1, emi_236/1
  cyemi_541/1 -> cfblk4/1
  cyemi_543/1 -> cfblk6/1
  cfblk3/1 -> cyemi_544/1, emi_420/1
  cfblk15/1 -> cyemi_545/1, emi_1860/1
  cfblk16/1 -> cyemi_546/1
  cfblk1/1 -> cyemi_547/1
  cyemi_544/1 -> cfblk7/1(emi_230)
  cyemi_545/1 -> cfblk7/2(emi_231)
  cfblk7/1(emi_232) -> cyemi_542/1
  emi_235/1 -> cfblk7/Action
  emi_235/2 -> emi_233/Action
  emi_236/1 -> emi_235/1
  cyemi_535/1 -> cfblk10/1(emi_415)
  cfblk10/1(emi_416) -> cyemi_541/1, cyemi_539/1
  emi_419/1 -> cfblk10/Action
  emi_419/2 -> emi_417/Action
  emi_420/1 -> emi_419/1
  cyemi_542/1 -> cfblk5/1(emi_995)
  cfblk5/1(emi_996) -> cyemi_543/1
  emi_999/1 -> cfblk5/Action
  emi_999/2 -> emi_997/Action
  emi_1000/1 -> emi_999/1
  cyemi_546/1 -> cfblk8/1(emi_1718)
  cfblk8/1(emi_1719) -> cyemi_535/1
  emi_1722/1 -> cfblk8/Action
  emi_1722/2 -> emi_1720/Action
  emi_1723/1 -> emi_1722/1
  cyemi_547/1 -> cfblk9/1(emi_1855)
  cfblk9/1(emi_1856) -> cyemi_537/1, cfblk14/1
  emi_1859/1 -> cfblk9/Action
  emi_1859/2 -> emi_1857/Action
  emi_1860/1 -> emi_1859/1

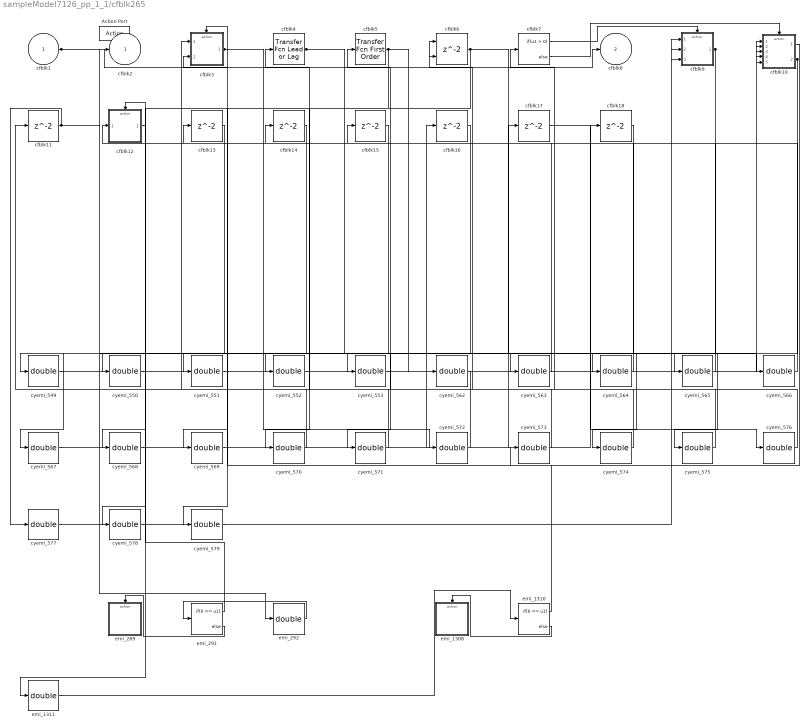
== system sampleModel7126_pp_1_1/cfblk265 ==
  cfblk1 : Inport
  Action Port : ActionPort  ActionType=then
  cfblk10 : Subsystem  TreatAsAtomicUnit=on
  cfblk{11,13..18} (7 alike) : Delay
  cfblk12 : Subsystem  TreatAsAtomicUnit=on
  cfblk3 : Subsystem  TreatAsAtomicUnit=on
  cfblk4 : simulink/Discrete/Transfer Fcn Lead or Lag  PoleZ=0.95  ZeroZ=0.75  ICPrevOutput=0.0  ICPrevInput=0.0  DoSatur=off
      settings: SourceProductName=Simulink  SourceProductBaseCode=SL
  cfblk5 : simulink/Discrete/Transfer Fcn First Order  PoleZ=0.95  ICPrevOutput=0.0  DoSatur=off
      settings: SourceProductName=Simulink
  cfblk6 : Delay  ShowEnablePort=on
      settings: InputPortMap=u0,e6
  cfblk7 : If  SampleTime=1
  cfblk9 : Subsystem  TreatAsAtomicUnit=on
  cyemi_{549..553,562..579} (23 alike) : DataTypeConversion  OutDataTypeStr=double
  emi_1308 : Subsystem  TreatAsAtomicUnit=on
  emi_1310 : If  IfExpression=0 <= u1  SampleTime=[1 0]
  emi_1311 : DataTypeConversion  OutDataTypeStr=double
  emi_289 : Subsystem  TreatAsAtomicUnit=on
  emi_291 : If  IfExpression=0 <= u1
  emi_292 : DataTypeConversion  OutDataTypeStr=double
  cfblk2 : Outport
  cfblk8 : Outport  Port=2
  wires:
  cfblk1/1 -> cfblk8/1, cfblk2/1, cyemi_553/1
  cfblk6/1 -> cyemi_566/1, cyemi_570/1, emi_1311/1
  cfblk10/2(cfblk15) -> cyemi_571/1, cyemi_575/1
  cfblk5/1 -> cyemi_562/1, cyemi_568/1, cyemi_569/1
  cfblk4/1 -> cyemi_563/1, cyemi_564/1
  cfblk9/1(cfblk2) -> cyemi_567/1, cyemi_574/1
  cfblk7/1 -> cfblk9/Action
  cfblk7/2 -> cfblk10/Action
  cyemi_549/1 -> cfblk10/1(cfblk1)
  cyemi_550/1 -> cfblk10/2(cfblk11)
  cfblk18/1 -> cyemi_550/1
  cyemi_551/1 -> cfblk10/3(cfblk12)
  cfblk14/1 -> cyemi_551/1
  cyemi_552/1 -> cfblk10/4(cfblk13)
  cfblk16/1 -> cyemi_552/1
  cyemi_553/1 -> cfblk10/5(cfblk14)
  cyemi_562/1 -> cfblk11/1
  cyemi_564/1 -> cfblk13/1
  cyemi_565/1 -> cfblk14/1
  cyemi_566/1 -> cfblk15/1
  cyemi_567/1 -> cfblk16/1
  cyemi_568/1 -> cfblk17/1
  cyemi_569/1 -> cfblk18/1
  cyemi_572/1 -> cfblk4/1
  cyemi_573/1 -> cfblk5/1
  cfblk10/1(cfblk2) -> cyemi_573/1
  cyemi_574/1 -> cfblk6/1
  cyemi_575/1 -> cfblk6/2
  cyemi_576/1 -> cfblk7/1
  cfblk17/1 -> cyemi_576/1
  cyemi_577/1 -> cfblk9/1(cfblk1)
  cfblk11/1 -> cyemi_577/1, emi_292/1
  cyemi_578/1 -> cfblk9/2(cfblk10)
  cfblk13/1 -> cyemi_578/1
  cyemi_579/1 -> cfblk9/3(cfblk11)
  cfblk15/1 -> cyemi_579/1
  cyemi_563/1 -> cfblk12/1(emi_287)
  cfblk12/1(emi_288) -> cyemi_549/1
  emi_291/1 -> cfblk12/Action
  emi_291/2 -> emi_289/Action
  emi_292/1 -> emi_291/1
  cyemi_570/1 -> cfblk3/1(emi_1305)
  cyemi_571/1 -> cfblk3/2(emi_1306)
  cfblk3/1(emi_1307) -> cyemi_572/1, cyemi_565/1
  emi_1310/1 -> cfblk3/Action
  emi_1310/2 -> emi_1308/Action
  emi_1311/1 -> emi_1310/1

== system sampleModel7126_pp_1_1/cfblk266 ==
  cfblk1 : Inport
  Action Port : ActionPort  ActionType=else
  cfblk10 : Subsystem  TreatAsAtomicUnit=on
  cfblk11 : Delay
  cfblk12 : Subsystem  TreatAsAtomicUnit=on
  cfblk13 : Delay
  cfblk14 : Subsystem  TreatAsAtomicUnit=on
  cfblk3 : Subsystem  TreatAsAtomicUnit=on
  cfblk4 : DiscreteIntegrator  SampleTime=-1  OutDataTypeStr=double  ICPrevOutput=DiscIntNeverNeededParam  ICPrevScaledInput=DiscIntNeverNeededParam
  cfblk5 : DiscreteTransferFcn
  cfblk6 : simulink/Continuous/PID Controller (2DOF)  Controller=PID  TimeDomain=Discrete-time  SampleTime=-1  IntegratorMethod=Forward Euler  FilterMethod=Forward Euler  Form=Parallel  UseFilter=on  ControllerParametersSource=internal  P=1  I=1  D=0  N=100  b=1  c=1  InitialConditionSource=internal  InitialConditionForIntegrator=0  InitialConditionForFilter=0  ExternalReset=none  LimitOutput=off  UpperSaturationLimit=inf  LowerSaturationLimit=-inf  LinearizeAsGain=off  AntiWindupMode=none  Kb=1  TrackingMode=off  Kt=1  PParamMin=[]  PParamMax=[]  IParamMin=[]  IParamMax=[]  DParamMin=[]  DParamMax=[]  NParamMin=[]  NParamMax=[]  bParamMin=[]  bParamMax=[]  cParamMin=[]  cParamMax=[]  KbParamMin=[]  KbParamMax=[]  KtParamMin=[]  KtParamMax=[]  POutMin=[]  POutMax=[]  IOutMin=[]  IOutMax=[]  DOutMin=[]  DOutMax=[]  NOutMin=[]  NOutMax=[]  bOutMin=[]  bOutMax=[]  cOutMin=[]  cOutMax=[]  KbOutMin=[]  KbOutMax=[]  KtOutMin=[]  KtOutMax=[]  IntegratorOutMin=[]  IntegratorOutMax=[]  FilterOutMin=[]  FilterOutMax=[]  SumOutMin=[]  SumOutMax=[]  Sum1OutMin=[]  Sum1OutMax=[]  Sum2OutMin=[]  Sum2OutMax=[]  Sum3OutMin=[]  Sum3OutMax=[]  SumI1OutMin=[]  SumI1OutMax=[]  SumI2OutMin=[]  SumI2OutMax=[]  SumI3OutMin=[]  SumI3OutMax=[]  SumDOutMin=[]  SumDOutMax=[]  SaturationOutMin=[]  SaturationOutMax=[]  IntegratorContinuousStateAttributes=''  IntegratorStateMustResolveToSignalObject=off  IntegratorRTWStateStorageClass=Auto  FilterContinuousStateAttributes=''  FilterStateMustResolveToSignalObject=off  FilterRTWStateStorageClass=Auto  DifferentiatorICPrevScaledInput=0  DifferentiatorOutMin=[]  DifferentiatorOutMax=[]  FilterDiffOutCoefMin=[]  FilterDiffOutCoefMax=[]  SumDenOutMin=[]  SumDenOutMax=[]  SumNumOutMin=[]  SumNumOutMax=[]  ReciprocalOutMin=[]  ReciprocalOutMax=[]  DivideOutMin=[]  DivideOutMax=[]  TunerSelectOption=Transfer Function Based (PID Tuner App)
  cfblk7 : DiscreteFilter
  cfblk8 : If  SampleTime=1
  cfblk9 : Subsystem  TreatAsAtomicUnit=on
  cyemi_{590,598..611} (15 alike) : DataTypeConversion  OutDataTypeStr=double
  emi_1226 : Subsystem  TreatAsAtomicUnit=on
  emi_1228 : If  IfExpression=0 <= u1  SampleTime=[1 0]
  emi_1229 : DataTypeConversion  OutDataTypeStr=double
  emi_1471 : Subsystem  TreatAsAtomicUnit=on
  emi_1473 : If  IfExpression=0 <= u1  SampleTime=[1 0]
  emi_1474 : DataTypeConversion  OutDataTypeStr=double
  emi_926 : Subsystem  TreatAsAtomicUnit=on
  emi_928 : If  IfExpression=0 <= u1
  emi_929 : DataTypeConversion  OutDataTypeStr=double
  cfblk2 : Outport
  wires:
  cfblk10/2(cfblk7) -> cfblk2/1
  cfblk4/1 -> cyemi_599/1, cyemi_600/1
  cfblk5/1 -> cyemi_590/1, cyemi_610/1
  cfblk8/1 -> cfblk9/Action
  cfblk8/2 -> cfblk10/Action
  cyemi_590/1 -> cfblk10/1(cfblk1)
  cyemi_598/1 -> cfblk11/1
  cfblk9/1(cfblk2) -> cyemi_598/1
  cyemi_600/1 -> cfblk13/1
  cfblk7/1 -> cyemi_601/1, emi_1229/1
  cfblk1/1 -> cyemi_602/1
  cyemi_603/1 -> cfblk4/1
  cfblk9/2(cfblk8) -> cyemi_603/1
  cyemi_604/1 -> cfblk5/1
  cyemi_605/1 -> cfblk6/1
  cfblk11/1 -> cyemi_605/1, emi_929/1
  cyemi_606/1 -> cfblk6/2
  cfblk10/1(cfblk2) -> cyemi_606/1
  cyemi_607/1 -> cfblk7/1
  cfblk6/1 -> cyemi_607/1
  cyemi_608/1 -> cfblk8/1
  cyemi_609/1 -> cfblk9/1(cfblk1)
  cyemi_610/1 -> cfblk9/2(cfblk6)
  cyemi_611/1 -> cfblk9/3(cfblk7)
  cfblk13/1 -> cyemi_611/1
  cyemi_599/1 -> cfblk12/1(emi_924)
  cfblk12/1(emi_925) -> cyemi_609/1, emi_1474/1
  emi_928/1 -> cfblk12/Action
  emi_928/2 -> emi_926/Action
  emi_929/1 -> emi_928/1
  cyemi_601/1 -> cfblk14/1(emi_1224)
  cfblk14/1(emi_1225) -> cyemi_608/1
  emi_1228/1 -> cfblk14/Action
  emi_1228/2 -> emi_1226/Action
  emi_1229/1 -> emi_1228/1
  cyemi_602/1 -> cfblk3/1(emi_1469)
  cfblk3/1(emi_1470) -> cyemi_604/1
  emi_1473/1 -> cfblk3/Action
  emi_1473/2 -> emi_1471/Action
  emi_1474/1 -> emi_1473/1

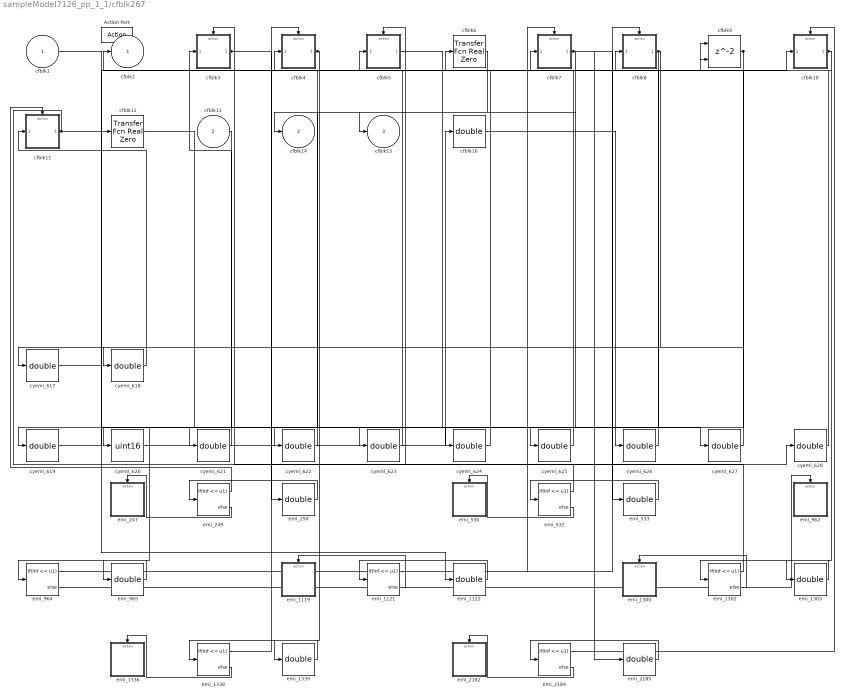
== system sampleModel7126_pp_1_1/cfblk267 ==
  cfblk1 : Inport
  cfblk13 : Inport  Port=2
  Action Port : ActionPort  ActionType=then
  cfblk10 : Subsystem  TreatAsAtomicUnit=on
  cfblk11 : Subsystem  TreatAsAtomicUnit=on
  cfblk12 : simulink/Discrete/Transfer Fcn Real Zero  ZeroZ=0.75  ICPrevInput=0.0  DoSatur=off
      settings: SourceProductName=Simulink  SourceProductBaseCode=SL
  cfblk16 : DataTypeConversion  OutDataTypeStr=double
  cfblk3 : Subsystem  TreatAsAtomicUnit=on
  cfblk4 : Subsystem  TreatAsAtomicUnit=on
  cfblk5 : Subsystem  TreatAsAtomicUnit=on
  cfblk6 : simulink/Discrete/Transfer Fcn Real Zero  ZeroZ=0.75  ICPrevInput=0.0  DoSatur=off
      settings: SourceProductName=Simulink  SourceProductBaseCode=SL
  cfblk7 : Subsystem  TreatAsAtomicUnit=on
  cfblk8 : Subsystem  TreatAsAtomicUnit=on
  cfblk9 : Delay  ShowEnablePort=on
      settings: InputPortMap=u0,e6
  cyemi_{617..619,621..628} (11 alike) : DataTypeConversion  OutDataTypeStr=double
  cyemi_620 : DataTypeConversion  OutDataTypeStr=uint16
  emi_1119 : Subsystem  TreatAsAtomicUnit=on
  emi_{249,532,964,1121,1302,1338} (6 alike) : If  IfExpression=Inf <= u1  SampleTime=[1 0]
  emi_{250,533,965,1122,1303,1339,2185} (7 alike) : DataTypeConversion  OutDataTypeStr=double
  emi_1300 : Subsystem  TreatAsAtomicUnit=on
  emi_1336 : Subsystem  TreatAsAtomicUnit=on
  emi_2182 : Subsystem  TreatAsAtomicUnit=on
  emi_2184 : If  IfExpression=Inf <= u1
  emi_247 : Subsystem  TreatAsAtomicUnit=on
  emi_530 : Subsystem  TreatAsAtomicUnit=on
  emi_962 : Subsystem  TreatAsAtomicUnit=on
  cfblk2 : Outport
  cfblk14 : Outport  Port=2
  cfblk15 : Outport  Port=3
  wires:
  cfblk9/1 -> cyemi_617/1, emi_965/1
  cyemi_619/1 -> cfblk12/1
  cyemi_620/1 -> cfblk16/1
  cfblk13/1 -> cyemi_620/1
  cfblk6/1 -> cyemi_622/1
  cfblk12/1 -> cyemi_623/1
  cyemi_624/1 -> cfblk6/1
  cfblk1/1 -> cyemi_624/1
  cfblk16/1 -> cyemi_626/1
  cyemi_627/1 -> cfblk9/1
  cyemi_628/1 -> cfblk9/2
  cyemi_618/1 -> cfblk11/1(emi_245)
  cfblk11/1(emi_246) -> cyemi_628/1, emi_1122/1
  emi_249/1 -> cfblk11/Action
  emi_249/2 -> emi_247/Action
  emi_250/1 -> emi_249/1
  cyemi_621/1 -> cfblk3/1(emi_528)
  cfblk3/1(emi_529) -> emi_250/1, cyemi_625/1
  emi_532/1 -> cfblk3/Action
  emi_532/2 -> emi_530/Action
  emi_533/1 -> emi_532/1
  cyemi_625/1 -> cfblk7/1(emi_960)
  cfblk7/1(emi_961) -> emi_533/1, cyemi_619/1, cfblk15/1, emi_2185/1
  emi_964/1 -> cfblk7/Action
  emi_964/2 -> emi_962/Action
  emi_965/1 -> emi_964/1
  cyemi_626/1 -> cfblk8/1(emi_1117)
  cfblk8/1(emi_1118) -> cyemi_618/1, emi_1339/1
  emi_1121/1 -> cfblk8/Action
  emi_1121/2 -> emi_1119/Action
  emi_1122/1 -> emi_1121/1
  cyemi_623/1 -> cfblk5/1(emi_1298)
  cfblk5/1(emi_1299) -> cyemi_627/1
  emi_1302/1 -> cfblk5/Action
  emi_1302/2 -> emi_1300/Action
  emi_1303/1 -> emi_1302/1
  cyemi_622/1 -> cfblk4/1(emi_1334)
  cfblk4/1(emi_1335) -> cyemi_621/1, cfblk14/1
  emi_1338/1 -> cfblk4/Action
  emi_1338/2 -> emi_1336/Action
  emi_1339/1 -> emi_1338/1
  cyemi_617/1 -> cfblk10/1(emi_2180)
  cfblk10/1(emi_2181) -> emi_1303/1, cfblk2/1
  emi_2184/1 -> cfblk10/Action
  emi_2184/2 -> emi_2182/Action
  emi_2185/1 -> emi_2184/1

== system sampleModel7126_pp_1_1/cfblk268 ==
  cfblk1 : Inport
  cfblk9 : Inport  Port=2
  cfblk10 : Inport  Port=3
  cfblk11 : Inport  Port=4
  Action Port : ActionPort  ActionType=else
  cfblk3 : Subsystem  TreatAsAtomicUnit=on
  cfblk4 : DiscreteIntegrator  SampleTime=-1  OutDataTypeStr=double  ICPrevOutput=DiscIntNeverNeededParam  ICPrevScaledInput=DiscIntNeverNeededParam
  cfblk5 : Subsystem  TreatAsAtomicUnit=on
  cfblk6 : DiscreteFir
  cfblk7 : Delay
  cfblk8 : Subsystem  TreatAsAtomicUnit=on
  cyemi_{633..638} (6 alike) : DataTypeConversion  OutDataTypeStr=double
  emi_1564 : Subsystem  TreatAsAtomicUnit=on
  emi_1566 : If  IfExpression=0 <= u1  SampleTime=[1 0]
  emi_1567 : DataTypeConversion  OutDataTypeStr=double
  emi_1691 : Subsystem  TreatAsAtomicUnit=on
  emi_1693 : If  IfExpression=0 <= u1  SampleTime=[1 0]
  emi_1694 : DataTypeConversion  OutDataTypeStr=double
  emi_642 : Subsystem  TreatAsAtomicUnit=on
  emi_644 : If  IfExpression=0 <= u1
  emi_645 : DataTypeConversion  OutDataTypeStr=double
  cfblk2 : Outport
  cfblk12 : Outport  Port=2
  cfblk13 : Outport  Port=3
  wires:
  cfblk4/1 -> cfblk13/1, emi_645/1, emi_1567/1
  cfblk6/1 -> cyemi_633/1
  cyemi_634/1 -> cfblk4/1
  cfblk10/1 -> cyemi_635/1
  cyemi_636/1 -> cfblk6/1
  cfblk7/1 -> cyemi_636/1, emi_1694/1
  cyemi_637/1 -> cfblk7/1
  cfblk1/1 -> cyemi_637/1
  cfblk9/1 -> cyemi_638/1
  cyemi_633/1 -> cfblk3/1(emi_640)
  cfblk3/1(emi_641) -> cfblk2/1
  emi_644/1 -> cfblk3/Action
  emi_644/2 -> emi_642/Action
  emi_645/1 -> emi_644/1
  cyemi_638/1 -> cfblk8/1(emi_1562)
  cfblk8/1(emi_1563) -> cfblk12/1
  emi_1566/1 -> cfblk8/Action
  emi_1566/2 -> emi_1564/Action
  emi_1567/1 -> emi_1566/1
  cyemi_635/1 -> cfblk5/1(emi_1689)
  cfblk5/1(emi_1690) -> cyemi_634/1
  emi_1693/1 -> cfblk5/Action
  emi_1693/2 -> emi_1691/Action
  emi_1694/1 -> emi_1693/1

== system sampleModel7126_pp_1_1/cfblk269 ==
  cfblk1 : Inport
  cfblk6 : Inport  Port=2
  Action Port : ActionPort  ActionType=then
  cfblk{10..13} (4 alike) : Delay
  cfblk14 : Subsystem  TreatAsAtomicUnit=on
  cfblk3 : Subsystem  TreatAsAtomicUnit=on
  cfblk4 : Subsystem  TreatAsAtomicUnit=on
  cfblk5 : If  SampleTime=1
  cfblk8 : Subsystem  TreatAsAtomicUnit=on
  cfblk9 : Subsystem  TreatAsAtomicUnit=on
  cyemi_{641..652,664..666} (15 alike) : DataTypeConversion  OutDataTypeStr=double
  emi_1742 : Subsystem  TreatAsAtomicUnit=on
  emi_1744 : If  IfExpression=Inf <= u1  SampleTime=[1 0]
  emi_1745 : DataTypeConversion  OutDataTypeStr=double
  emi_1779 : Subsystem  TreatAsAtomicUnit=on
  emi_1781 : If  IfExpression=Inf <= u1  SampleTime=[1 0]
  emi_1782 : DataTypeConversion  OutDataTypeStr=double
  emi_492 : Subsystem  TreatAsAtomicUnit=on
  emi_494 : If  IfExpression=Inf <= u1  SampleTime=[1 0]
  emi_495 : DataTypeConversion  OutDataTypeStr=double
  cfblk2 : Outport
  cfblk7 : Outport  Port=2
  wires:
  cfblk8/1(cfblk2) -> cfblk7/1
  cfblk6/1 -> cyemi_651/1, cyemi_666/1
  cfblk5/1 -> cfblk8/Action
  cfblk5/2 -> cfblk9/Action
  cyemi_641/1 -> cfblk10/1
  cyemi_642/1 -> cfblk11/1
  cfblk9/1(cfblk2) -> cyemi_642/1
  cyemi_643/1 -> cfblk12/1
  cyemi_644/1 -> cfblk13/1
  cfblk9/3(cfblk11) -> cyemi_644/1
  cfblk9/4(cfblk12) -> cyemi_645/1
  cfblk9/2(cfblk10) -> cyemi_646/1
  cfblk8/2(cfblk14) -> cyemi_647/1
  cfblk13/1 -> cyemi_648/1, emi_1745/1
  cyemi_649/1 -> cfblk5/1
  cfblk11/1 -> cyemi_649/1
  cyemi_650/1 -> cfblk8/1(cfblk1)
  cfblk1/1 -> cyemi_650/1
  cyemi_651/1 -> cfblk8/2(cfblk12)
  cyemi_652/1 -> cfblk8/3(cfblk13)
  cyemi_664/1 -> cfblk9/1(cfblk1)
  cfblk10/1 -> cyemi_664/1, emi_495/1, emi_1782/1
  cyemi_665/1 -> cfblk9/2(cfblk8)
  cfblk12/1 -> cyemi_665/1
  cyemi_666/1 -> cfblk9/3(cfblk9)
  cyemi_647/1 -> cfblk4/1(emi_489)
  cyemi_648/1 -> cfblk4/2(emi_490)
  cfblk4/1(emi_491) -> cyemi_641/1
  emi_494/1 -> cfblk4/Action
  emi_494/2 -> emi_492/Action
  emi_495/1 -> emi_494/1
  cyemi_645/1 -> cfblk14/1(emi_1740)
  cfblk14/1(emi_1741) -> cyemi_652/1
  emi_1744/1 -> cfblk14/Action
  emi_1744/2 -> emi_1742/Action
  emi_1745/1 -> emi_1744/1
  cyemi_646/1 -> cfblk3/1(emi_1777)
  cfblk3/1(emi_1778) -> cyemi_643/1, cfblk2/1
  emi_1781/1 -> cfblk3/Action
  emi_1781/2 -> emi_1779/Action
  emi_1782/1 -> emi_1781/1
